simulink model "PI_s"  (R2023a)
settings: Solver=VariableStepAuto  StartTime=0.0  StopTime=10.0  RelTol=1e-3
undefined symbols (not defined in the file): DiscIntNeverNeededParam, Kaw, Ki, Kp, Tdref_ay_bp_ms2, Tdref_table, Tdref_v_bp_ms, Ts_ctrl
settings Model: Creator=Tan_Tram  LastModifiedBy=Tan_Tram

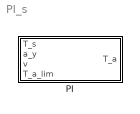
== system PI_s ==
  PI : Subsystem

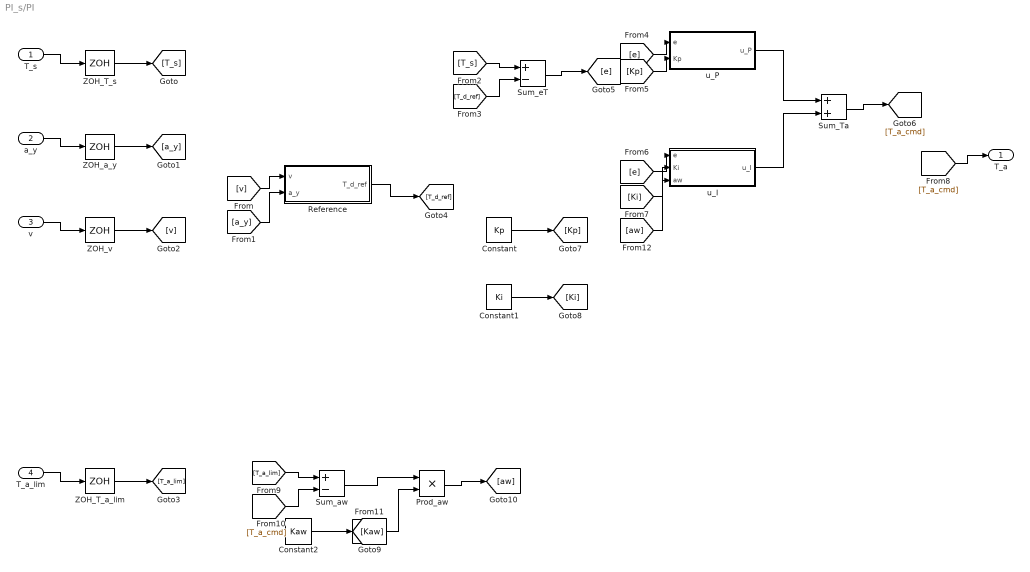
== system PI_s/PI ==
  T_s : Inport
  a_y : Inport  Port=2
  v : Inport  Port=3
  T_a_lim : Inport  Port=4
  Constant : Constant  Value=Kp
  Constant1 : Constant  Value=Ki
  Constant2 : Constant  Value=Kaw
  Prod_aw : Product  Inputs=**
  Reference : Subsystem
  Sum_Ta : Sum
  Sum_aw : Sum  Inputs=+-
  Sum_eT : Sum  Inputs=+-
  ZOH_T_a_lim : ZeroOrderHold  SampleTime=Ts_ctrl
  ZOH_T_s : ZeroOrderHold  SampleTime=Ts_ctrl
  ZOH_a_y : ZeroOrderHold  SampleTime=Ts_ctrl
  ZOH_v : ZeroOrderHold  SampleTime=Ts_ctrl
  u_I : Subsystem
  u_P : Subsystem
  T_a : Outport
  wires:
  T_s/1 -> ZOH_T_s/1
  ZOH_T_s/1 -> [T_s]
  a_y/1 -> ZOH_a_y/1
  ZOH_a_y/1 -> [a_y]
  v/1 -> ZOH_v/1
  ZOH_v/1 -> [v]
  T_a_lim/1 -> ZOH_T_a_lim/1
  ZOH_T_a_lim/1 -> [T_a_lim]
  [v] -> Reference/1(v)
  [a_y] -> Reference/2(a_y)
  Reference/1(T_d_ref) -> [T_d_ref]
  [T_s] -> Sum_eT/1
  [T_d_ref] -> Sum_eT/2
  Sum_eT/1 -> [e]
  [e] -> u_P/1(e)
  [Kp] -> u_P/2(Kp)
  [e] -> u_I/1(e)
  [Ki] -> u_I/2(Ki)
  u_P/1(u_P) -> Sum_Ta/1
  u_I/1(u_I) -> Sum_Ta/2
  Sum_Ta/1 -> [T_a_cmd]
  [T_a_cmd] -> T_a/1
  [T_a_lim] -> Sum_aw/1
  [T_a_cmd] -> Sum_aw/2
  Sum_aw/1 -> Prod_aw/1
  [Kaw] -> Prod_aw/2
  Constant/1 -> [Kp]
  Constant1/1 -> [Ki]
  Constant2/1 -> [Kaw]
  Prod_aw/1 -> [aw]
  [aw] -> u_I/3(aw)

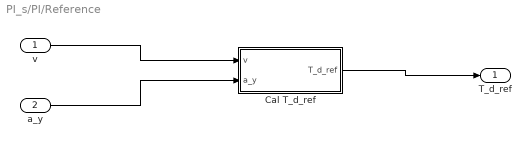
== system PI_s/PI/Reference ==
  v : Inport
  a_y : Inport  Port=2
  Cal T_d_ref : Subsystem
  T_d_ref : Outport
  wires:
  Cal T_d_ref/1(T_d_ref) -> T_d_ref/1
  a_y/1 -> Cal T_d_ref/2(a_y)
  v/1 -> Cal T_d_ref/1(v)

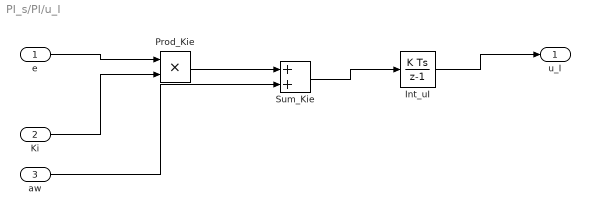
== system PI_s/PI/u_I ==
  e : Inport
  Ki : Inport  Port=2
  aw : Inport  Port=3
  Int_uI : DiscreteIntegrator  SampleTime=Ts_ctrl  ICPrevOutput=DiscIntNeverNeededParam  ICPrevScaledInput=DiscIntNeverNeededParam
  Prod_Kie : Product  Inputs=**
  Sum_Kie : Sum
  u_I : Outport
  wires:
  e/1 -> Prod_Kie/1
  Ki/1 -> Prod_Kie/2
  Prod_Kie/1 -> Sum_Kie/1
  aw/1 -> Sum_Kie/2
  Sum_Kie/1 -> Int_uI/1
  Int_uI/1 -> u_I/1

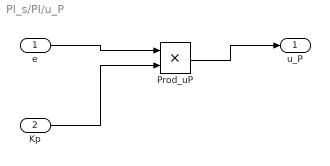
== system PI_s/PI/u_P ==
  e : Inport
  Kp : Inport  Port=2
  Prod_uP : Product  Inputs=**
  u_P : Outport
  wires:
  e/1 -> Prod_uP/1
  Kp/1 -> Prod_uP/2
  Prod_uP/1 -> u_P/1

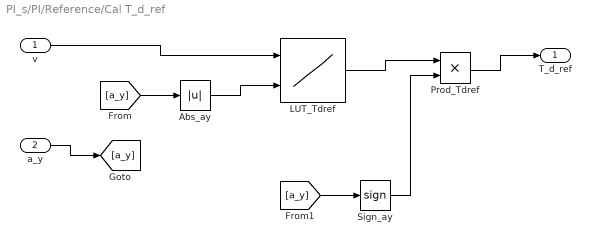
== system PI_s/PI/Reference/Cal T_d_ref ==
  v : Inport
  a_y : Inport  Port=2
  Abs_ay : Abs  SaturateOnIntegerOverflow=off
  LUT_Tdref : Lookup_n-D  BreakpointsForDimension1=Tdref_v_bp_ms  BreakpointsForDimension2=Tdref_ay_bp_ms2  Table=Tdref_table  ExtrapMethod=Clip  InternalRulePriority=Speed  RndMeth=Simplest
      settings: InputPortMap=u0,u1
  Prod_Tdref : Product  Inputs=**
  Sign_ay : Signum
  T_d_ref : Outport
  wires:
  Prod_Tdref/1 -> T_d_ref/1
  Sign_ay/1 -> Prod_Tdref/2
  LUT_Tdref/1 -> Prod_Tdref/1
  [a_y] -> Sign_ay/1
  Abs_ay/1 -> LUT_Tdref/2
  [a_y] -> Abs_ay/1
  v/1 -> LUT_Tdref/1
  a_y/1 -> [a_y]
